simulink model "boot_demo"  (Simulink 7.3)
settings: Solver=FixedStepDiscrete  SolverMode=SingleTasking  StartTime=0.0  StopTime=10.0  RelTol=1e-3
PreLoadFcn:
  | waijung.modelPreload; % Required for working with Waijung Blockset. Do not remove.
undefined symbols (not defined in the file): HSEOSC, Link, LQFP176, ST, STM32F417IG
libraries: simulink x43, stm32f4_flash_lib x14, waijung_filestream_lib x4, stm32f4_crc_lib x3, stm32f4_boot_lib x2, stm32f4_io_lib x1, stm32f4_reset_lib x1, stm32f4_device_config_lib x1
CloseFcn:
  | waijung.modelClose; % Required for working with Waijung Blockset. Do not remove.
settings Model: Creator=Krisada  LastModifiedBy=Krisada
settings OptimizationCC: OptimizeModelRefInitCode=on  LifeSpan=1
settings HardwareCC: ProdEndianess=LittleEndian  ProdHWDeviceType=ARM Compatible->Cortex - M4  TargetEndianess=LittleEndian  TargetHWDeviceType=ARM Compatible->Cortex - M4
settings RTWCC: SystemTargetFile=stm32f4.tlc  GenerateMakefile=off  TemplateMakefile=ert_default_tmf  Description=STM32F4 Target  ProcessScript=stm32f4_make_rtw_hook
settings CodeAppCC: IgnoreCustomStorageClasses=off
settings STFCustomTargetCC: ModelReferenceCompliant=off  CombineOutputUpdateFcns=on  ERTCustomFileBanners=on  SupportContinuousTime=off  SupportNonInlinedSFcns=off  SystemTargetFile=stm32f4.tlc
settings ERTTargetCC: MultiwordLength=2048  ModelReferenceCompliant=off  ParMdlRefBuildCompliant=off  CompOptLevelCompliant=off  ERTFirstTimeCompliant=off  ModelStepFunctionPrototypeControlCompliant=off  CPPClassGenCompliant=off  ExtModeMexFile=noextcomm  InlinedParameterPlacement=NonHierarchical  ERTSrcFileBannerTemplate=stm32f4_code_template.cgt  ERTHdrFileBannerTemplate=stm32f4_code_template.cgt  ERTDataSrcFileTemplate=stm32f4_code_template.cgt  ERTDataHdrFileTemplate=stm32f4_code_template.cgt  ERTCustomFileTemplate=stm32f4_file_process.tlc

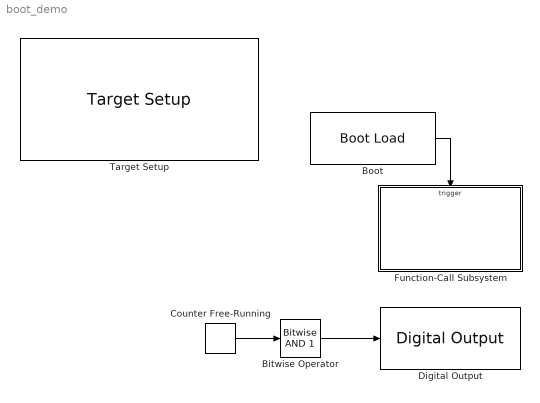
== system boot_demo ==
  Bitwise Operator : simulink/Logic and Bit Operations/Bitwise Operator  logicop=AND  UseBitMask=on  BitMask=1  BitMaskRealWorld=Stored Integer
  Boot : stm32f4_boot_lib/Boot Load  conf=Boot  flashorigin=0x8000000  flashlength=0x100000  enableisr=on  usersector=Sector 9: 0x080A0000 - 0x080BFFFF  sampletime=-1  sampletimestr=0.01  blockid=Boot  inputarray=[]  inputlabelarray={}  outputarray=[7]  outputlabelarray={'Call ISR'}  compat=0  confstr="[\"080A0000\",\"9\"]"
  Counter Free-Running : simulink/Sources/Counter Free-Running  SystemSampleTime=-1  NumBits=16  tsamp=0.5
  Digital Output : stm32f4_io_lib/Digital Output  use_bitband=on  port=D  speed=100  porttype=Push Pull  porttypestr=PP  use_pin0=off  use_pin1=off  use_pin2=off  use_pin3=off  use_pin4=off  use_pin5=off  use_pin6=off  use_pin7=off  use_pin8=off  use_pin9=off  use_pin10=off  use_pin11=off  use_pin12=off  use_pin13=off  use_pin14=off  use_pin15=on  pinstr=GPIO_Pin_15  usedpinarray="[0  0  0  0  0  0  0  0  0  0  0  0  0  0  0  1]"  bitbandingstr="#define DigitalOutput_D15 Peripheral_BB(GPIOD->ODR, 15)  /* Output pin */"  sampletime=-1  sampletimestr=0.5  blockid=DigitalOutput  enablecustomportlabel=off  globalinit=off  cinputportlabel=In1, In2  coutputportlabel=0
  Function-Call Subsystem : Subsystem  TreatAsAtomicUnit=on
  Target Setup : stm32f4_device_config_lib/Target Setup  Priority=100  compiler=GNU ARM  previous_compiler=GNU ARM  mcu=STM32F417IG (LQFP176)  mcustr=STM32F417IG  clockconfig=HSEOSC-8MHz  system_stm32f4xx_c_path=F:\trunk\targets\stm32f4_target\stm32f4\utils\system_stm32f4xx_default\STM32F40_41xxx\hseosc8mhz  showmemoryconfiguration=off  stacksize=0x2000  heapsize=0x2000  enableautocompiledownload=on  fullchiperase=on  programmerinterface=ST-Link  editctrlstr=on  compilercontrolstr=$(patsubst %, -I%, .) -mcpu=cortex-m4 -mthumb -mthumb-interwork -mfloat-abi=hard -mfpu=fpv4-sp-d16 -ffast-math -Wall -Wextra -Ofast  assemblercontrolstr=$(patsubst %, -I%, .) -mcpu=cortex-m4 -mthumb -mthumb-interwork -mfloat-abi=hard -mfpu=fpv4-sp-d16 -ffast-math -Wall -Wextra -Ofast -Wa,-amhls=$(<:.s=.lst) -D__STACK_SIZE=$(STACK_SIZE) -D__HEAP_SIZE=$(HEAP_SIZE)  linkercontrolstr=-T$(LD_SCRIPT) -g -Wl,-Map=$(MAP),--cref,--no-warn-mismatch -mcpu=cortex-m4 -mthumb -mthumb-interwork -mfloat-abi=hard -mfpu=fpv4-sp-d16 -specs=nosys.specs  runafterdownload=on  execprofile=None  profileruart=3  profilerbaud=500000  profilertxpin=D8  profilerinitstr=0.01,168000000,1680000,500000,0  manualsetsampletime=off  sampletime=0.01  blockid=TargetSetup  systickreloadvalue=1680000  hseval=8000000  lastprofileruart=3  hclk=168000000  flashorigin=0x8000000  flashlength=1024k  ramorigin=0x20000000  ramlength=128k  useextram=off
  wires:
  Boot/1 -> Function-Call Subsystem/Trigger
  Counter Free-Running/1 -> Bitwise Operator/1
  Bitwise Operator/1 -> Digital Output/1

== system boot_demo/Function-Call Subsystem ==
  function : TriggerPort  TriggerType=function-call
  Load system/conf.ini : Subsystem  TreatAsAtomicUnit=on
  Logical Operator1 : Logic  Operator=NOT  AllPortsSameDT=off  OutDataTypeMode=boolean  LogicDataType=fixdt(0, 8)  OutDataTypeStr=boolean
  System Upgrade : Subsystem
  Validate Main Program : Subsystem
  wires:
  Load system/conf.ini/1(Upgrade Enable) -> System Upgrade/Enable, Logical Operator1/1
  Load system/conf.ini/2(File) -> System Upgrade/1(File)
  Logical Operator1/1 -> Validate Main Program/Enable

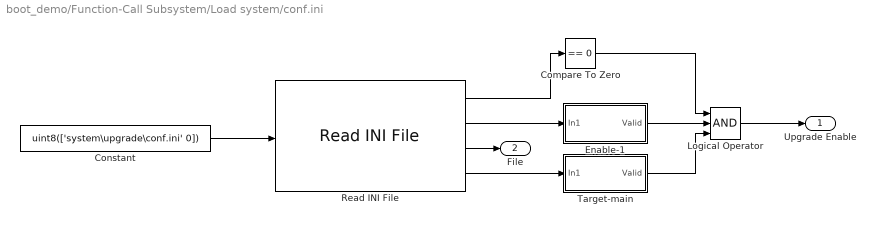
== system boot_demo/Function-Call Subsystem/Load system/conf.ini ==
  Compare To Zero : simulink/Logic and Bit Operations/Compare To Zero  SystemSampleTime=-1  relop===  LogicOutDataTypeMode=uint8  ZeroCross=off
  Constant : Constant  Value=uint8(['system\upgrade\conf.ini' 0])  OutDataType=fixdt(1, 16)  OutScaling=2^0
  Enable-1 : Subsystem
  Logical Operator : Logic  Inputs=3  AllPortsSameDT=off  OutDataTypeMode=boolean  LogicDataType=fixdt(0, 8)  OutDataTypeStr=boolean
  Read INI File : waijung_filestream_lib/Read INI File  conf=INIRead  inisection='Upgrade'  inikeys={'Enable','File','Target'}  datatype=double  datacount=1  maxstring=128  valuetype=Vector  portpinstr=0  sampletime=inf  blockid=FunctionCallSubsystemLoadsystemconfiniReadINIFile  inputporttype=[-1]  inputportwidth=[-1]  inputportlabel={'FilePath'}  outputporttype=[6 3 3 3]  outputportwidth=[1 128 128 128]  outputportlabel={'Status' 'Enable' 'File' 'Target'}  compat=0  optionstring="[\"Upgrade\",\"128\"]"  inikeylist="[\"Enable\",\"File\",\"Target\"]"
  Target-main : Subsystem
  Upgrade Enable : Outport  OutDataType=fixdt(1, 16)  OutScaling=2^0
  File : Outport  Port=2  OutDataType=fixdt(1, 16)  OutScaling=2^0
  wires:
  Constant/1 -> Read INI File/1
  Read INI File/3 -> File/1
  Read INI File/2 -> Enable-1/1(In1)
  Read INI File/4 -> Target-main/1(In1)
  Target-main/1(Valid) -> Logical Operator/3
  Enable-1/1(Valid) -> Logical Operator/2
  Read INI File/1 -> Compare To Zero/1
  Logical Operator/1 -> Upgrade Enable/1
  Compare To Zero/1 -> Logical Operator/1

== system boot_demo/Function-Call Subsystem/System Upgrade ==
  File : Inport  OutDataType=fixdt(1, 16)  OutScaling=2^0
  Enable : EnablePort
  Add : Sum  Inputs=+++  OutDataType=fixdt(1, 16)  OutScaling=2^-10
  Clear system/conf.ini : Subsystem
  Upgrade : Subsystem  TreatAsAtomicUnit=on
  Validate File : Subsystem  TreatAsAtomicUnit=on
  Verify : Subsystem  TreatAsAtomicUnit=on
  wires:
  Validate File/1(Update File Valid) -> Upgrade/Enable, Add/1
  File/1 -> Validate File/1(File), Upgrade/1(File), Clear system/conf.ini/2(File)
  Upgrade/1(Success) -> Verify/Enable, Add/2
  Verify/1(Success) -> Add/3
  Add/1 -> Clear system/conf.ini/1(Success State)

== system boot_demo/Function-Call Subsystem/Validate Main Program ==
  Enable : EnablePort
  CRC Location : Constant  Value=uint32(hex2dec('20000')-4)  OutDataType=fixdt(1, 16)  OutScaling=2^0
  Flash Read : stm32f4_flash_lib/Flash Read  conf=Read  transfer=Blocking  flashsector=Sector 7: 0x08060000 - 0x0807FFFF  datatype=uint32  datacount=1  enablestatus=off  sampletime=-1  sampletimestr=-1  blockid=FunctionCallSubsystemValidateMainProgramFlashRead  inputarray=[-1]  inputlabelarray={'Offset '}  outputarray=[7]  outputlabelarray={'Data (uint32)'}  compat=0  confstr="[\"uint32\",\"20000\",\"08060000\",\"7\",\"off\"]"
  JumpToSectorB : Subsystem  TreatAsAtomicUnit=on
  Relational Operator : RelationalOperator  Operator===  LogicOutDataTypeMode=boolean  LogicDataType=fixdt(0, 8)  OutDataTypeStr=boolean
  While Iterator Subsystem1 : Subsystem  TreatAsAtomicUnit=on
  wires:
  Flash Read/1 -> Relational Operator/1
  While Iterator Subsystem1/1(Sector CRC) -> Relational Operator/2
  CRC Location/1 -> Flash Read/1
  Relational Operator/1 -> JumpToSectorB/Enable

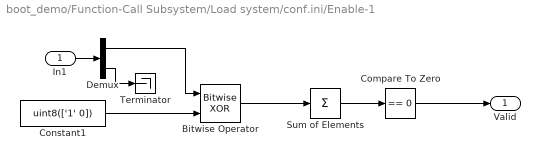
== system boot_demo/Function-Call Subsystem/Load system/conf.ini/Enable-1 ==
  In1 : Inport
  Bitwise Operator : simulink/Logic and Bit Operations/Bitwise Operator  logicop=XOR  UseBitMask=off  NumInputPorts=2  BitMask=bin2dec('11011001')  BitMaskRealWorld=Stored Integer
  Compare To Zero : simulink/Logic and Bit Operations/Compare To Zero  SystemSampleTime=-1  relop===  LogicOutDataTypeMode=uint8  ZeroCross=off
  Constant1 : Constant  Value=uint8(['1' 0])  OutDataType=fixdt(1, 16)  OutScaling=2^0
  Demux : Demux  Outputs=[2 -1]
  Sum of Elements : Sum  Inputs=+  OutDataType=fixdt(1, 16)  OutScaling=2^-10
  Terminator : Terminator
  Valid : Outport
  wires:
  In1/1 -> Demux/1
  Constant1/1 -> Bitwise Operator/2
  Bitwise Operator/1 -> Sum of Elements/1
  Sum of Elements/1 -> Compare To Zero/1
  Compare To Zero/1 -> Valid/1
  Demux/2 -> Terminator/1
  Demux/1 -> Bitwise Operator/1

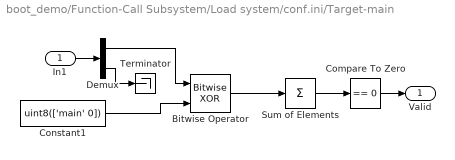
== system boot_demo/Function-Call Subsystem/Load system/conf.ini/Target-main ==
  In1 : Inport
  Bitwise Operator : simulink/Logic and Bit Operations/Bitwise Operator  logicop=XOR  UseBitMask=off  NumInputPorts=2  BitMask=bin2dec('11011001')  BitMaskRealWorld=Stored Integer
  Compare To Zero : simulink/Logic and Bit Operations/Compare To Zero  SystemSampleTime=-1  relop===  LogicOutDataTypeMode=uint8  ZeroCross=off
  Constant1 : Constant  Value=uint8(['main' 0])  OutDataType=fixdt(1, 16)  OutScaling=2^0
  Demux : Demux  Outputs=[5 -1]
  Sum of Elements : Sum  Inputs=+  OutDataType=fixdt(1, 16)  OutScaling=2^-10
  Terminator : Terminator
  Valid : Outport
  wires:
  Constant1/1 -> Bitwise Operator/2
  In1/1 -> Demux/1
  Bitwise Operator/1 -> Sum of Elements/1
  Sum of Elements/1 -> Compare To Zero/1
  Compare To Zero/1 -> Valid/1
  Demux/2 -> Terminator/1
  Demux/1 -> Bitwise Operator/1

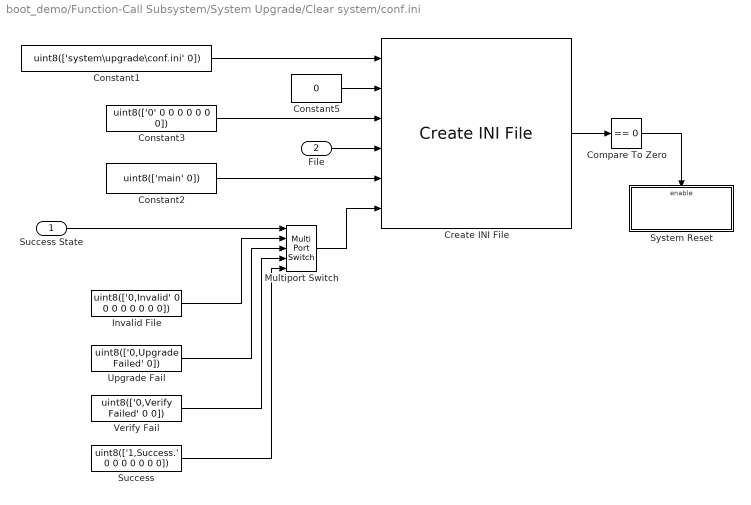
== system boot_demo/Function-Call Subsystem/System Upgrade/Clear system/conf.ini ==
  Success State : Inport  OutDataType=fixdt(1, 16)  OutScaling=2^0
  File : Inport  Port=2  OutDataType=fixdt(1, 16)  OutScaling=2^0
  Compare To Zero : simulink/Logic and Bit Operations/Compare To Zero  SystemSampleTime=-1  relop===  LogicOutDataTypeMode=uint8  ZeroCross=off
  Constant1 : Constant  Value=uint8(['system\upgrade\conf.ini' 0])  OutDataType=fixdt(1, 16)  OutScaling=2^0
  Constant2 : Constant  Value=uint8(['main' 0])  OutDataType=fixdt(1, 16)  OutScaling=2^0
  Constant3 : Constant  Value=uint8(['0' 0 0 0 0 0 0 0])  OutDataType=fixdt(1, 16)  OutScaling=2^0
  Constant5 : Constant  Value=0  OutDataType=fixdt(1, 16)  OutScaling=2^0
  Create INI File : waijung_filestream_lib/Create INI File  conf=INICreate  inisection='Upgrade'  inikeys={'Enable','File','Target','Status'}  datatype=double  datacount=1  maxstring=32  valuetype=Pointer  portpinstr=0  sampletime=inf  blockid=FunctionCallSubsystemSystemUpgradeClearsystemconfiniCreateINIFile  inputporttype=[-1 -1 -1 -1 -1 -1]  inputportwidth=[-1 1 -1 -1 -1 -1]  inputportlabel={'FilePath','Append' 'Enable' 'File' 'Target' 'Status'}  outputporttype=[6]  outputportwidth=[]  outputportlabel={'Status'}  compat=0  optionstring="[\"Upgrade\",\"32\"]"  inikeylist="[\"Enable\",\"File\",\"Target\",\"Status\"]"
  Invalid File : Constant  Value=uint8(['0,Invalid' 0 0 0 0 0 0 0 0])  OutDataType=fixdt(1, 16)  OutScaling=2^0
  Multiport Switch : MultiPortSwitch  Inputs=4  zeroidx=on  OutDataType=fixdt(1, 16)  OutScaling=2^0
  Success : Constant  Value=uint8(['1,Success.' 0 0 0 0 0 0 0])  OutDataType=fixdt(1, 16)  OutScaling=2^0
  System Reset : Subsystem  TreatAsAtomicUnit=on
  Upgrade Fail : Constant  Value=uint8(['0,Upgrade Failed' 0])  OutDataType=fixdt(1, 16)  OutScaling=2^0
  Verify Fail : Constant  Value=uint8(['0,Verify Failed' 0 0])  OutDataType=fixdt(1, 16)  OutScaling=2^0
  wires:
  Constant3/1 -> Create INI File/3
  Constant1/1 -> Create INI File/1
  Create INI File/1 -> Compare To Zero/1
  Compare To Zero/1 -> System Reset/Enable
  Success State/1 -> Multiport Switch/1
  Multiport Switch/1 -> Create INI File/6
  Constant2/1 -> Create INI File/5
  File/1 -> Create INI File/4
  Constant5/1 -> Create INI File/2
  Invalid File/1 -> Multiport Switch/2
  Upgrade Fail/1 -> Multiport Switch/3
  Verify Fail/1 -> Multiport Switch/4
  Success/1 -> Multiport Switch/5

== system boot_demo/Function-Call Subsystem/System Upgrade/Upgrade ==
  File : Inport  OutDataType=fixdt(1, 16)  OutScaling=2^0
  Enable : EnablePort
  Copy New Program : Subsystem  TreatAsAtomicUnit=on
  Erase Main Program Sector : Subsystem
  Success : Outport  OutDataType=fixdt(1, 16)  OutScaling=2^0
  wires:
  Erase Main Program Sector/1(Erased) -> Copy New Program/Enable
  File/1 -> Copy New Program/1(File)
  Copy New Program/1(Success) -> Success/1

== system boot_demo/Function-Call Subsystem/System Upgrade/Validate File ==
  File : Inport  OutDataType=fixdt(1, 16)  OutScaling=2^0
  Logical Operator : Logic  AllPortsSameDT=off  OutDataTypeMode=boolean  LogicDataType=fixdt(0, 8)  OutDataTypeStr=boolean
  Relational Operator : RelationalOperator  Operator===  LogicOutDataTypeMode=boolean  LogicDataType=fixdt(0, 8)  OutDataTypeStr=boolean
  While Iterator Subsystem : Subsystem  TreatAsAtomicUnit=on
  Update File Valid : Outport  OutDataType=fixdt(1, 16)  OutScaling=2^0
  wires:
  File/1 -> While Iterator Subsystem/1(File)
  While Iterator Subsystem/2(File CRC) -> Relational Operator/1
  While Iterator Subsystem/3(Emb CRC) -> Relational Operator/2
  Relational Operator/1 -> Logical Operator/2
  While Iterator Subsystem/1(Success) -> Logical Operator/1
  Logical Operator/1 -> Update File Valid/1

== system boot_demo/Function-Call Subsystem/System Upgrade/Verify ==
  Enable : EnablePort
  CRC Location : Constant  Value=uint32(hex2dec('20000')-4)  OutDataType=fixdt(1, 16)  OutScaling=2^0
  Flash Read : stm32f4_flash_lib/Flash Read  conf=Read  transfer=Blocking  flashsector=Sector 7: 0x08060000 - 0x0807FFFF  datatype=uint32  datacount=1  enablestatus=off  sampletime=-1  sampletimestr=-1  blockid=FunctionCallSubsystemSystemUpgradeVerifyFlashRead  inputarray=[-1]  inputlabelarray={'Offset '}  outputarray=[7]  outputlabelarray={'Data (uint32)'}  compat=0  confstr="[\"uint32\",\"20000\",\"08060000\",\"7\",\"off\"]"
  Relational Operator : RelationalOperator  Operator===  LogicOutDataTypeMode=boolean  LogicDataType=fixdt(0, 8)  OutDataTypeStr=boolean
  While Iterator Subsystem1 : Subsystem  TreatAsAtomicUnit=on
  Success : Outport  OutDataType=fixdt(1, 16)  OutScaling=2^0
  wires:
  Flash Read/1 -> Relational Operator/1
  While Iterator Subsystem1/1(Sector CRC) -> Relational Operator/2
  CRC Location/1 -> Flash Read/1
  Relational Operator/1 -> Success/1

== system boot_demo/Function-Call Subsystem/Validate Main Program/JumpToSectorB ==
  Enable : EnablePort
  Boot : stm32f4_boot_lib/Jump Sector  conf=Goto  flashorigin=0x8000000  flashlength=0x100000  enableisr=off  usersector=Sector 5: 0x08020000 - 0x0803FFFF  sampletime=inf  sampletimestr=-1  blockid=FunctionCallSubsystemValidateMainProgramJumpToSectorBBoot  inputarray=[]  inputlabelarray={}  outputarray=[]  outputlabelarray={}  compat=0  confstr="[\"08020000\",\"5\"]"

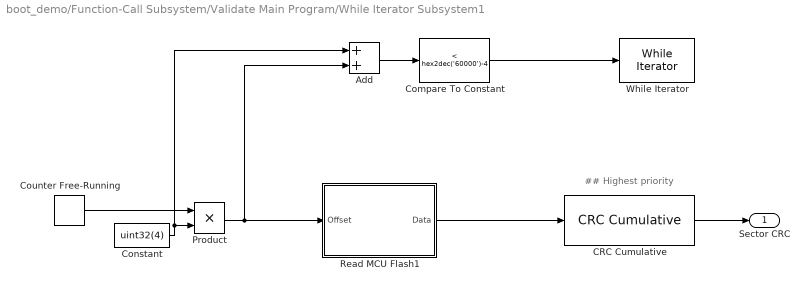
== system boot_demo/Function-Call Subsystem/Validate Main Program/While Iterator Subsystem1 ==
  note: ## Highest priority
  Add : Sum  OutDataType=fixdt(1, 16)  OutScaling=2^-10
  CRC Cumulative : stm32f4_crc_lib/CRC Cumulative  Priority=0  conf=Cumulative  sampletime=-1  sampletimestr=-1  blockid=FunctionCallSubsystemValidateMainProgramWhileIteratorSubsystem1CRCCumulative  inputarray=[7]  inputlabelarray={'uint32'}  outputarray=[7]  outputlabelarray={'uint32'}  compat=0  confstr="[\"Param1\",\"Param1\"]"
  Compare To Constant : simulink/Logic and Bit Operations/Compare To Constant  SystemSampleTime=-1  relop=<  const=hex2dec('60000')-4  LogicOutDataTypeMode=uint8  ZeroCross=off
  Constant : Constant  Value=uint32(4)  OutDataType=fixdt(1, 16)  OutScaling=2^0
  Counter Free-Running : simulink/Sources/Counter Free-Running  SystemSampleTime=-1  NumBits=32  tsamp=-1
  Product : Product  OutDataTypeMode=uint32  OutDataType=fixdt(1, 16)  OutScaling=2^0  OutDataTypeStr=uint32  RndMeth=Zero
  Read MCU Flash1 : Subsystem
  While Iterator : WhileIterator  Priority=1  MaxIters=-1  WhileBlockType=do-while
  Sector CRC : Outport  OutDataType=fixdt(1, 16)  OutScaling=2^0
  wires:
  Counter Free-Running/1 -> Product/1
  Compare To Constant/1 -> While Iterator/1
  Product/1 -> Add/2, Read MCU Flash1/1(Offset)
  Constant/1 -> Product/2, Add/1
  Read MCU Flash1/1(Data) -> CRC Cumulative/1
  CRC Cumulative/1 -> Sector CRC/1
  Add/1 -> Compare To Constant/1

== system boot_demo/Function-Call Subsystem/System Upgrade/Clear system/conf.ini/System Reset ==
  Enable : EnablePort
  System Reset : stm32f4_reset_lib/System Reset  conf=<empty>  sampletime=inf  sampletimestr=-1  blockid=FunctionCallSubsystemSystemUpgradeClearsystemconfiniSystemResetSystemReset  inputarray=[]  inputlabelarray={}  outputarray=[]  outputlabelarray={}  compat=0  confstr="[\"Param1\",\"Param1\"]"

== system boot_demo/Function-Call Subsystem/System Upgrade/Upgrade/Copy New Program ==
  File : Inport  OutDataType=fixdt(1, 16)  OutScaling=2^0
  Enable : EnablePort
  Read File-Write Flash : Subsystem  TreatAsAtomicUnit=on
  Success : Outport  OutDataType=fixdt(1, 16)  OutScaling=2^0
  wires:
  File/1 -> Read File-Write Flash/1(File)
  Read File-Write Flash/1(Success) -> Success/1

== system boot_demo/Function-Call Subsystem/System Upgrade/Upgrade/Erase Main Program Sector ==
  Compare To Zero : simulink/Logic and Bit Operations/Compare To Zero  SystemSampleTime=-1  relop===  LogicOutDataTypeMode=uint8  ZeroCross=off
  Compare To Zero1 : simulink/Logic and Bit Operations/Compare To Zero  SystemSampleTime=-1  relop===  LogicOutDataTypeMode=uint8  ZeroCross=off
  Compare To Zero2 : simulink/Logic and Bit Operations/Compare To Zero  SystemSampleTime=-1  relop===  LogicOutDataTypeMode=uint8  ZeroCross=off
  Flash Erase : stm32f4_flash_lib/Flash Erase  conf=Erase  transfer=Blocking  flashsector=Sector 5: 0x08020000 - 0x0803FFFF  datatype=uint32  datacount=1  enablestatus=on  sampletime=-1  sampletimestr=-1  blockid=FunctionCallSubsystemSystemUpgradeUpgradeEraseMainProgramSectorFlashErase  inputarray=[]  inputlabelarray={}  outputarray=[3]  outputlabelarray={'Status'}  compat=0  confstr="[\"Blocking\",\"on\",\"08020000\",\"5\"]"
  Flash Erase1 : stm32f4_flash_lib/Flash Erase  conf=Erase  transfer=Blocking  flashsector=Sector 6: 0x08040000 - 0x0805FFFF  datatype=uint32  datacount=1  enablestatus=on  sampletime=-1  sampletimestr=-1  blockid=FunctionCallSubsystemSystemUpgradeUpgradeEraseMainProgramSectorFlashErase1  inputarray=[]  inputlabelarray={}  outputarray=[3]  outputlabelarray={'Status'}  compat=0  confstr="[\"Blocking\",\"on\",\"08040000\",\"6\"]"
  Flash Erase2 : stm32f4_flash_lib/Flash Erase  conf=Erase  transfer=Blocking  flashsector=Sector 7: 0x08060000 - 0x0807FFFF  datatype=uint32  datacount=1  enablestatus=on  sampletime=-1  sampletimestr=-1  blockid=FunctionCallSubsystemSystemUpgradeUpgradeEraseMainProgramSectorFlashErase2  inputarray=[]  inputlabelarray={}  outputarray=[3]  outputlabelarray={'Status'}  compat=0  confstr="[\"Blocking\",\"on\",\"08060000\",\"7\"]"
  Logical Operator : Logic  Inputs=3  AllPortsSameDT=off  OutDataTypeMode=boolean  LogicDataType=fixdt(0, 8)  OutDataTypeStr=boolean
  Erased : Outport  OutDataType=fixdt(1, 16)  OutScaling=2^0
  wires:
  Flash Erase/1 -> Compare To Zero/1
  Flash Erase1/1 -> Compare To Zero1/1
  Flash Erase2/1 -> Compare To Zero2/1
  Compare To Zero1/1 -> Logical Operator/2
  Compare To Zero/1 -> Logical Operator/1
  Compare To Zero2/1 -> Logical Operator/3
  Logical Operator/1 -> Erased/1

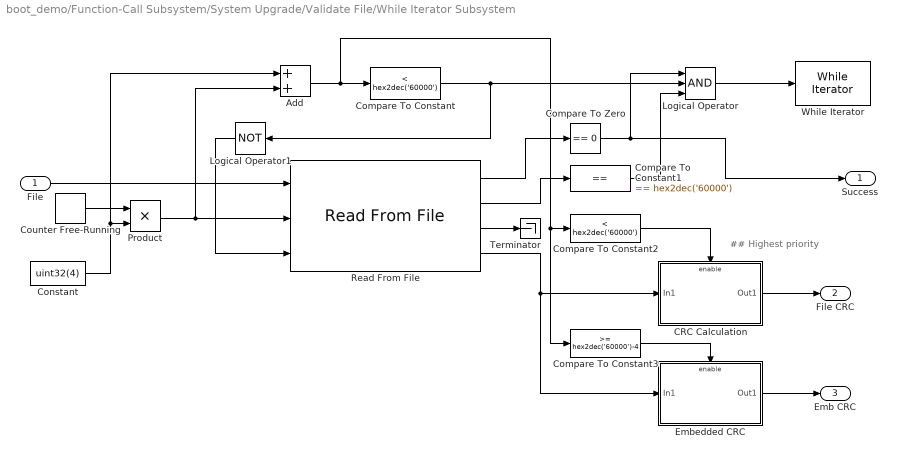
== system boot_demo/Function-Call Subsystem/System Upgrade/Validate File/While Iterator Subsystem ==
  note: ## Highest priority
  File : Inport  OutDataType=fixdt(1, 16)  OutScaling=2^0
  Add : Sum  OutDataType=fixdt(1, 16)  OutScaling=2^-10
  CRC Calculation : Subsystem
  Compare To Constant : simulink/Logic and Bit Operations/Compare To Constant  SystemSampleTime=-1  relop=<  const=hex2dec('60000')  LogicOutDataTypeMode=uint8  ZeroCross=off
  Compare To Constant1 : simulink/Logic and Bit Operations/Compare To Constant  SystemSampleTime=-1  relop===  const=hex2dec('60000')  LogicOutDataTypeMode=uint8  ZeroCross=off
  Compare To Constant2 : simulink/Logic and Bit Operations/Compare To Constant  SystemSampleTime=-1  relop=<  const=hex2dec('60000')  LogicOutDataTypeMode=uint8  ZeroCross=off
  Compare To Constant3 : simulink/Logic and Bit Operations/Compare To Constant  SystemSampleTime=-1  relop=>=  const=hex2dec('60000')-4  LogicOutDataTypeMode=uint8  ZeroCross=off
  Compare To Zero : simulink/Logic and Bit Operations/Compare To Zero  SystemSampleTime=-1  relop===  LogicOutDataTypeMode=uint8  ZeroCross=off
  Constant : Constant  Value=uint32(4)  OutDataType=fixdt(1, 16)  OutScaling=2^0
  Counter Free-Running : simulink/Sources/Counter Free-Running  SystemSampleTime=-1  NumBits=32  tsamp=-1
  Embedded CRC : Subsystem
  Logical Operator : Logic  Inputs=3  AllPortsSameDT=off  OutDataTypeMode=boolean  LogicDataType=fixdt(0, 8)  OutDataTypeStr=boolean
  Logical Operator1 : Logic  Operator=NOT  AllPortsSameDT=off  OutDataTypeMode=boolean  LogicDataType=fixdt(0, 8)  OutDataTypeStr=boolean
  Product : Product  OutDataTypeMode=uint32  OutDataType=fixdt(1, 16)  OutScaling=2^0  OutDataTypeStr=uint32  RndMeth=Zero
  Read From File : waijung_filestream_lib/Read From File  conf=ReadFromFile  inisection='Boot'  inikeys={'Action','File'}  datatype=uint32  datacount=1  maxstring=32  valuetype=Pointer  portpinstr=0  sampletime=inf  blockid=FunctionCallSubsystemSystemUpgradeValidateFileWhileIteratorSubsystemReadFromFile  inputporttype=[-1 -1 -1]  inputportwidth=[-1 1 1]  inputportlabel={'FilePath','SeekPos','Close'}  outputporttype=[6 7 7 7]  outputportwidth=[1 1 1 1]  outputportlabel={'Status','TotalSize','CurrentPos','Data (uint32)'}  compat=0  optionstring="[\"Boot\",\"32\"]"  inikeylist="[\"Action\",\"File\"]"
  Terminator : Terminator
  While Iterator : WhileIterator  Priority=1  MaxIters=-1  WhileBlockType=do-while
  Success : Outport  OutDataType=fixdt(1, 16)  OutScaling=2^0
  File CRC : Outport  Port=2  OutDataType=fixdt(1, 16)  OutScaling=2^0
  Emb CRC : Outport  Port=3  OutDataType=fixdt(1, 16)  OutScaling=2^0
  wires:
  Counter Free-Running/1 -> Product/1
  Constant/1 -> Product/2, Add/1
  CRC Calculation/1(Out1) -> File CRC/1
  Add/1 -> Compare To Constant/1, Compare To Constant2/1, Compare To Constant3/1
  Read From File/4 -> CRC Calculation/1(In1), Embedded CRC/1(In1)
  File/1 -> Read From File/1
  Read From File/2 -> Compare To Constant1/1
  Read From File/1 -> Compare To Zero/1
  Logical Operator/1 -> While Iterator/1
  Compare To Constant/1 -> Logical Operator/2, Logical Operator1/1
  Compare To Zero/1 -> Logical Operator/1, Success/1
  Compare To Constant1/1 -> Logical Operator/3
  Read From File/3 -> Terminator/1
  Product/1 -> Read From File/2, Add/2
  Compare To Constant2/1 -> CRC Calculation/Enable
  Compare To Constant3/1 -> Embedded CRC/Enable
  Embedded CRC/1(Out1) -> Emb CRC/1
  Logical Operator1/1 -> Read From File/3

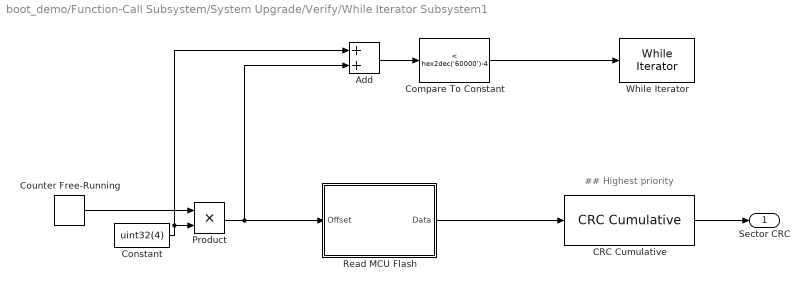
== system boot_demo/Function-Call Subsystem/System Upgrade/Verify/While Iterator Subsystem1 ==
  note: ## Highest priority
  Add : Sum  OutDataType=fixdt(1, 16)  OutScaling=2^-10
  CRC Cumulative : stm32f4_crc_lib/CRC Cumulative  Priority=0  conf=Cumulative  sampletime=-1  sampletimestr=-1  blockid=FunctionCallSubsystemSystemUpgradeVerifyWhileIteratorSubsystem1CRCCumulative  inputarray=[7]  inputlabelarray={'uint32'}  outputarray=[7]  outputlabelarray={'uint32'}  compat=0  confstr="[\"Param1\",\"Param1\"]"
  Compare To Constant : simulink/Logic and Bit Operations/Compare To Constant  SystemSampleTime=-1  relop=<  const=hex2dec('60000')-4  LogicOutDataTypeMode=uint8  ZeroCross=off
  Constant : Constant  Value=uint32(4)  OutDataType=fixdt(1, 16)  OutScaling=2^0
  Counter Free-Running : simulink/Sources/Counter Free-Running  SystemSampleTime=-1  NumBits=32  tsamp=-1
  Product : Product  OutDataTypeMode=uint32  OutDataType=fixdt(1, 16)  OutScaling=2^0  OutDataTypeStr=uint32  RndMeth=Zero
  Read MCU Flash : Subsystem
  While Iterator : WhileIterator  Priority=1  MaxIters=-1  WhileBlockType=do-while
  Sector CRC : Outport  OutDataType=fixdt(1, 16)  OutScaling=2^0
  wires:
  Counter Free-Running/1 -> Product/1
  Compare To Constant/1 -> While Iterator/1
  Product/1 -> Add/2, Read MCU Flash/1(Offset)
  Constant/1 -> Product/2, Add/1
  Read MCU Flash/1(Data) -> CRC Cumulative/1
  CRC Cumulative/1 -> Sector CRC/1
  Add/1 -> Compare To Constant/1

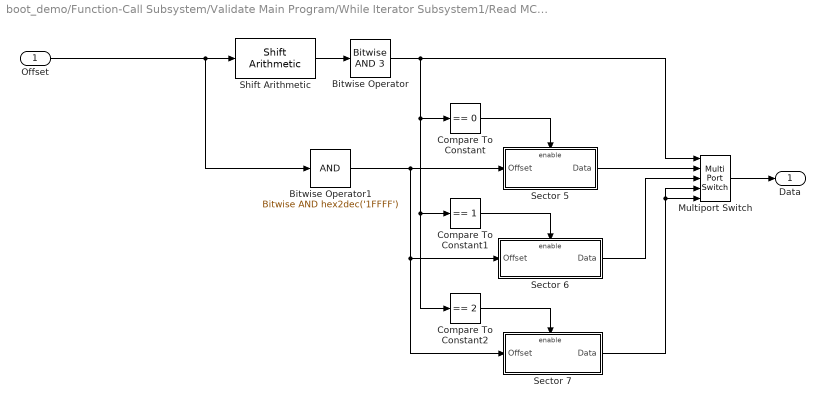
== system boot_demo/Function-Call Subsystem/Validate Main Program/While Iterator Subsystem1/Read MCU Flash1 ==
  Offset : Inport
  Bitwise Operator : simulink/Logic and Bit Operations/Bitwise Operator  logicop=AND  UseBitMask=on  BitMask=3  BitMaskRealWorld=Stored Integer
  Bitwise Operator1 : simulink/Logic and Bit Operations/Bitwise Operator  logicop=AND  UseBitMask=on  BitMask=hex2dec('1FFFF')  BitMaskRealWorld=Stored Integer
  Compare To Constant : simulink/Logic and Bit Operations/Compare To Constant  SystemSampleTime=-1  relop===  const=0  LogicOutDataTypeMode=uint8  ZeroCross=off
  Compare To Constant1 : simulink/Logic and Bit Operations/Compare To Constant  SystemSampleTime=-1  relop===  const=1  LogicOutDataTypeMode=uint8  ZeroCross=off
  Compare To Constant2 : simulink/Logic and Bit Operations/Compare To Constant  SystemSampleTime=-1  relop===  const=2  LogicOutDataTypeMode=uint8  ZeroCross=off
  Multiport Switch : MultiPortSwitch  Inputs=4  zeroidx=on  OutDataType=fixdt(1, 16)  OutScaling=2^0
  Sector 5 : Subsystem  TreatAsAtomicUnit=on
  Sector 6 : Subsystem  TreatAsAtomicUnit=on
  Sector 7 : Subsystem  TreatAsAtomicUnit=on
  Shift Arithmetic : simulink/Logic and Bit Operations/Shift Arithmetic  SystemSampleTime=-1  nBitShiftRight=17  nBinPtShiftRight=0
  Data : Outport
  wires:
  Sector 7/1(Data) -> Multiport Switch/5, Multiport Switch/4
  Sector 6/1(Data) -> Multiport Switch/3
  Bitwise Operator1/1 -> Sector 7/1(Offset), Sector 6/1(Offset), Sector 5/1(Offset)
  Offset/1 -> Bitwise Operator1/1, Shift Arithmetic/1
  Multiport Switch/1 -> Data/1
  Sector 5/1(Data) -> Multiport Switch/2
  Compare To Constant2/1 -> Sector 7/Enable
  Compare To Constant1/1 -> Sector 6/Enable
  Compare To Constant/1 -> Sector 5/Enable
  Bitwise Operator/1 -> Multiport Switch/1, Compare To Constant2/1, Compare To Constant1/1, Compare To Constant/1
  Shift Arithmetic/1 -> Bitwise Operator/1

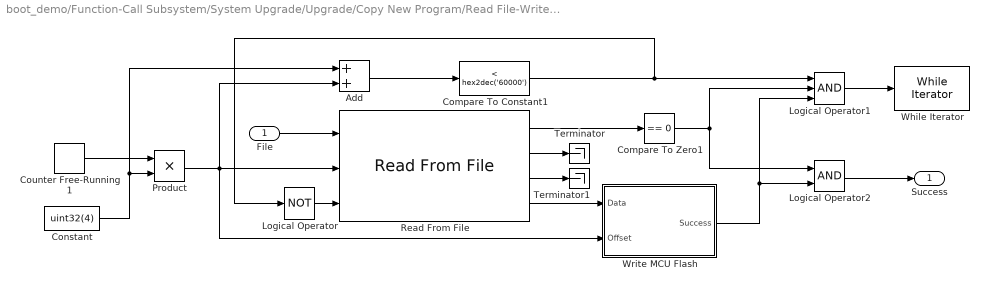
== system boot_demo/Function-Call Subsystem/System Upgrade/Upgrade/Copy New Program/Read File-Write Flash ==
  File : Inport  OutDataType=fixdt(1, 16)  OutScaling=2^0
  Add : Sum  OutDataType=fixdt(1, 16)  OutScaling=2^-10
  Compare To Constant1 : simulink/Logic and Bit Operations/Compare To Constant  SystemSampleTime=-1  relop=<  const=hex2dec('60000')  LogicOutDataTypeMode=uint8  ZeroCross=off
  Compare To Zero1 : simulink/Logic and Bit Operations/Compare To Zero  SystemSampleTime=-1  relop===  LogicOutDataTypeMode=uint8  ZeroCross=off
  Constant : Constant  Value=uint32(4)  OutDataType=fixdt(1, 16)  OutScaling=2^0
  Counter Free-Running1 : simulink/Sources/Counter Free-Running  SystemSampleTime=-1  NumBits=32  tsamp=-1
  Logical Operator : Logic  Operator=NOT  AllPortsSameDT=off  OutDataTypeMode=boolean  LogicDataType=fixdt(0, 8)  OutDataTypeStr=boolean
  Logical Operator1 : Logic  Inputs=3  AllPortsSameDT=off  OutDataTypeMode=boolean  LogicDataType=fixdt(0, 8)  OutDataTypeStr=boolean
  Logical Operator2 : Logic  AllPortsSameDT=off  OutDataTypeMode=boolean  LogicDataType=fixdt(0, 8)  OutDataTypeStr=boolean
  Product : Product  OutDataTypeMode=uint32  OutDataType=fixdt(1, 16)  OutScaling=2^0  OutDataTypeStr=uint32  RndMeth=Zero
  Read From File : waijung_filestream_lib/Read From File  conf=ReadFromFile  inisection='Boot'  inikeys={'Action','File'}  datatype=uint32  datacount=1  maxstring=32  valuetype=Pointer  portpinstr=0  sampletime=inf  blockid=FunctionCallSubsystemSystemUpgradeUpgradeCopyNewProgramReadFileWriteFlashReadFromFile  inputporttype=[-1 -1 -1]  inputportwidth=[-1 1 1]  inputportlabel={'FilePath','SeekPos','Close'}  outputporttype=[6 7 7 7]  outputportwidth=[1 1 1 1]  outputportlabel={'Status','TotalSize','CurrentPos','Data (uint32)'}  compat=0  optionstring="[\"Boot\",\"32\"]"  inikeylist="[\"Action\",\"File\"]"
  Terminator : Terminator
  Terminator1 : Terminator
  While Iterator : WhileIterator  MaxIters=-1  WhileBlockType=do-while
  Write MCU Flash : Subsystem
  Success : Outport  OutDataType=fixdt(1, 16)  OutScaling=2^0
  wires:
  Logical Operator1/1 -> While Iterator/1
  Compare To Constant1/1 -> Logical Operator1/1, Logical Operator/1
  Add/1 -> Compare To Constant1/1
  Constant/1 -> Add/1, Product/2
  Product/1 -> Add/2, Read From File/2, Write MCU Flash/2(Offset)
  Counter Free-Running1/1 -> Product/1
  File/1 -> Read From File/1
  Logical Operator/1 -> Read From File/3
  Read From File/1 -> Compare To Zero1/1
  Compare To Zero1/1 -> Logical Operator1/2, Logical Operator2/1
  Read From File/4 -> Write MCU Flash/1(Data)
  Logical Operator2/1 -> Success/1
  Read From File/2 -> Terminator/1
  Read From File/3 -> Terminator1/1
  Write MCU Flash/1(Success) -> Logical Operator2/2, Logical Operator1/3

== system boot_demo/Function-Call Subsystem/System Upgrade/Validate File/While Iterator Subsystem/CRC Calculation ==
  In1 : Inport
  Enable : EnablePort
  CRC Cumulative : stm32f4_crc_lib/CRC Cumulative  Priority=0  conf=Cumulative  sampletime=-1  sampletimestr=-1  blockid=FunctionCallSubsystemSystemUpgradeValidateFileWhileIteratorSubsystemCRCCalculationCRCCumulative  inputarray=[7]  inputlabelarray={'uint32'}  outputarray=[7]  outputlabelarray={'uint32'}  compat=0  confstr="[\"Param1\",\"Param1\"]"
  Out1 : Outport
  wires:
  In1/1 -> CRC Cumulative/1
  CRC Cumulative/1 -> Out1/1

== system boot_demo/Function-Call Subsystem/System Upgrade/Validate File/While Iterator Subsystem/Embedded CRC ==
  In1 : Inport
  Enable : EnablePort
  Out1 : Outport
  wires:
  In1/1 -> Out1/1

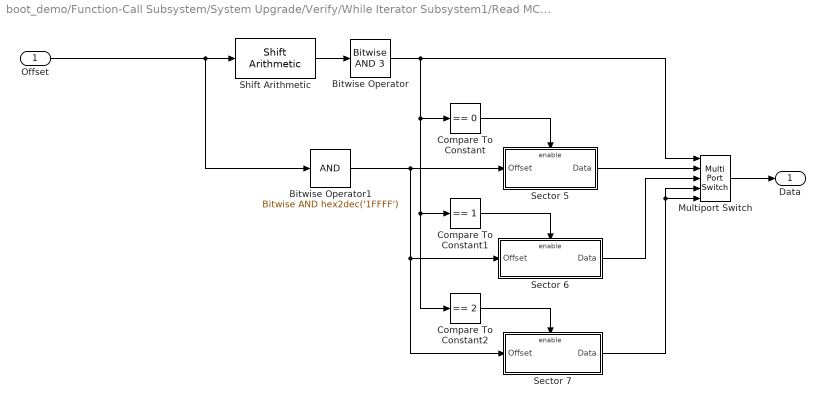
== system boot_demo/Function-Call Subsystem/System Upgrade/Verify/While Iterator Subsystem1/Read MCU Flash ==
  Offset : Inport
  Bitwise Operator : simulink/Logic and Bit Operations/Bitwise Operator  logicop=AND  UseBitMask=on  BitMask=3  BitMaskRealWorld=Stored Integer
  Bitwise Operator1 : simulink/Logic and Bit Operations/Bitwise Operator  logicop=AND  UseBitMask=on  BitMask=hex2dec('1FFFF')  BitMaskRealWorld=Stored Integer
  Compare To Constant : simulink/Logic and Bit Operations/Compare To Constant  SystemSampleTime=-1  relop===  const=0  LogicOutDataTypeMode=uint8  ZeroCross=off
  Compare To Constant1 : simulink/Logic and Bit Operations/Compare To Constant  SystemSampleTime=-1  relop===  const=1  LogicOutDataTypeMode=uint8  ZeroCross=off
  Compare To Constant2 : simulink/Logic and Bit Operations/Compare To Constant  SystemSampleTime=-1  relop===  const=2  LogicOutDataTypeMode=uint8  ZeroCross=off
  Multiport Switch : MultiPortSwitch  Inputs=4  zeroidx=on  OutDataType=fixdt(1, 16)  OutScaling=2^0
  Sector 5 : Subsystem  TreatAsAtomicUnit=on
  Sector 6 : Subsystem  TreatAsAtomicUnit=on
  Sector 7 : Subsystem  TreatAsAtomicUnit=on
  Shift Arithmetic : simulink/Logic and Bit Operations/Shift Arithmetic  SystemSampleTime=-1  nBitShiftRight=17  nBinPtShiftRight=0
  Data : Outport
  wires:
  Shift Arithmetic/1 -> Bitwise Operator/1
  Bitwise Operator/1 -> Compare To Constant/1, Compare To Constant1/1, Compare To Constant2/1, Multiport Switch/1
  Compare To Constant/1 -> Sector 5/Enable
  Compare To Constant1/1 -> Sector 6/Enable
  Compare To Constant2/1 -> Sector 7/Enable
  Sector 5/1(Data) -> Multiport Switch/2
  Multiport Switch/1 -> Data/1
  Offset/1 -> Shift Arithmetic/1, Bitwise Operator1/1
  Bitwise Operator1/1 -> Sector 5/1(Offset), Sector 6/1(Offset), Sector 7/1(Offset)
  Sector 6/1(Data) -> Multiport Switch/3
  Sector 7/1(Data) -> Multiport Switch/4, Multiport Switch/5

== system boot_demo/Function-Call Subsystem/Validate Main Program/While Iterator Subsystem1/Read MCU Flash1/Sector 5 ==
  Offset : Inport  OutDataType=fixdt(1, 16)  OutScaling=2^0
  Enable : EnablePort
  Flash Read : stm32f4_flash_lib/Flash Read  conf=Read  transfer=Blocking  flashsector=Sector 5: 0x08020000 - 0x0803FFFF  datatype=uint32  datacount=1  enablestatus=on  sampletime=-1  sampletimestr=-1  blockid=FunctionCallSubsystemValidateMainProgramWhileIteratorSubsystem1ReadMCUFlash1Sector5FlashRead  inputarray=[-1]  inputlabelarray={'Offset '}  outputarray=[7]  outputlabelarray={'Data (uint32)'}  compat=0  confstr="[\"uint32\",\"20000\",\"08020000\",\"5\",\"on\"]"
  Data : Outport  OutDataType=fixdt(1, 16)  OutScaling=2^0
  wires:
  Flash Read/1 -> Data/1
  Offset/1 -> Flash Read/1

== system boot_demo/Function-Call Subsystem/Validate Main Program/While Iterator Subsystem1/Read MCU Flash1/Sector 6 ==
  Offset : Inport  OutDataType=fixdt(1, 16)  OutScaling=2^0
  Enable : EnablePort
  Flash Read : stm32f4_flash_lib/Flash Read  conf=Read  transfer=Blocking  flashsector=Sector 6: 0x08040000 - 0x0805FFFF  datatype=uint32  datacount=1  enablestatus=on  sampletime=-1  sampletimestr=-1  blockid=FunctionCallSubsystemValidateMainProgramWhileIteratorSubsystem1ReadMCUFlash1Sector6FlashRead  inputarray=[-1]  inputlabelarray={'Offset '}  outputarray=[7]  outputlabelarray={'Data (uint32)'}  compat=0  confstr="[\"uint32\",\"20000\",\"08040000\",\"6\",\"on\"]"
  Data : Outport  OutDataType=fixdt(1, 16)  OutScaling=2^0
  wires:
  Offset/1 -> Flash Read/1
  Flash Read/1 -> Data/1

== system boot_demo/Function-Call Subsystem/Validate Main Program/While Iterator Subsystem1/Read MCU Flash1/Sector 7 ==
  Offset : Inport  OutDataType=fixdt(1, 16)  OutScaling=2^0
  Enable : EnablePort
  Flash Read : stm32f4_flash_lib/Flash Read  conf=Read  transfer=Blocking  flashsector=Sector 7: 0x08060000 - 0x0807FFFF  datatype=uint32  datacount=1  enablestatus=on  sampletime=-1  sampletimestr=-1  blockid=FunctionCallSubsystemValidateMainProgramWhileIteratorSubsystem1ReadMCUFlash1Sector7FlashRead  inputarray=[-1]  inputlabelarray={'Offset '}  outputarray=[7]  outputlabelarray={'Data (uint32)'}  compat=0  confstr="[\"uint32\",\"20000\",\"08060000\",\"7\",\"on\"]"
  Data : Outport  OutDataType=fixdt(1, 16)  OutScaling=2^0
  wires:
  Offset/1 -> Flash Read/1
  Flash Read/1 -> Data/1

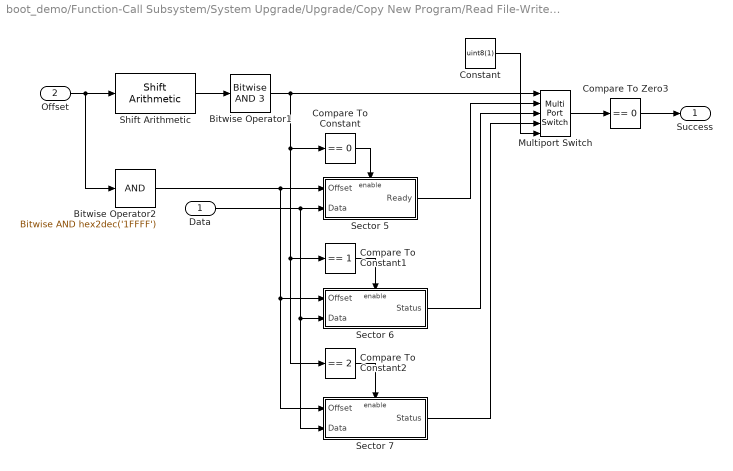
== system boot_demo/Function-Call Subsystem/System Upgrade/Upgrade/Copy New Program/Read File-Write Flash/Write MCU Flash ==
  Data : Inport
  Offset : Inport  Port=2
  Bitwise Operator1 : simulink/Logic and Bit Operations/Bitwise Operator  logicop=AND  UseBitMask=on  BitMask=3  BitMaskRealWorld=Stored Integer
  Bitwise Operator2 : simulink/Logic and Bit Operations/Bitwise Operator  logicop=AND  UseBitMask=on  BitMask=hex2dec('1FFFF')  BitMaskRealWorld=Stored Integer
  Compare To Constant : simulink/Logic and Bit Operations/Compare To Constant  SystemSampleTime=-1  relop===  const=0  LogicOutDataTypeMode=uint8  ZeroCross=off
  Compare To Constant1 : simulink/Logic and Bit Operations/Compare To Constant  SystemSampleTime=-1  relop===  const=1  LogicOutDataTypeMode=uint8  ZeroCross=off
  Compare To Constant2 : simulink/Logic and Bit Operations/Compare To Constant  SystemSampleTime=-1  relop===  const=2  LogicOutDataTypeMode=uint8  ZeroCross=off
  Compare To Zero3 : simulink/Logic and Bit Operations/Compare To Zero  SystemSampleTime=-1  relop===  LogicOutDataTypeMode=uint8  ZeroCross=off
  Constant : Constant  Value=uint8(1)  OutDataType=fixdt(1, 16)  OutScaling=2^0
  Multiport Switch : MultiPortSwitch  Inputs=4  zeroidx=on  OutDataType=fixdt(1, 16)  OutScaling=2^0
  Sector 5 : Subsystem  TreatAsAtomicUnit=on
  Sector 6 : Subsystem  TreatAsAtomicUnit=on
  Sector 7 : Subsystem  TreatAsAtomicUnit=on
  Shift Arithmetic : simulink/Logic and Bit Operations/Shift Arithmetic  SystemSampleTime=-1  nBitShiftRight=17  nBinPtShiftRight=0
  Success : Outport
  wires:
  Shift Arithmetic/1 -> Bitwise Operator1/1
  Offset/1 -> Shift Arithmetic/1, Bitwise Operator2/1
  Compare To Constant/1 -> Sector 5/Enable
  Bitwise Operator1/1 -> Compare To Constant/1, Compare To Constant1/1, Compare To Constant2/1, Multiport Switch/1
  Bitwise Operator2/1 -> Sector 5/1(Offset), Sector 6/1(Offset), Sector 7/1(Offset)
  Data/1 -> Sector 5/2(Data), Sector 6/2(Data), Sector 7/2(Data)
  Compare To Constant1/1 -> Sector 6/Enable
  Compare To Constant2/1 -> Sector 7/Enable
  Multiport Switch/1 -> Compare To Zero3/1
  Compare To Zero3/1 -> Success/1
  Sector 5/1(Ready) -> Multiport Switch/2
  Sector 6/1(Status) -> Multiport Switch/3
  Sector 7/1(Status) -> Multiport Switch/4
  Constant/1 -> Multiport Switch/5

== system boot_demo/Function-Call Subsystem/System Upgrade/Verify/While Iterator Subsystem1/Read MCU Flash/Sector 5 ==
  Offset : Inport  OutDataType=fixdt(1, 16)  OutScaling=2^0
  Enable : EnablePort
  Flash Read : stm32f4_flash_lib/Flash Read  conf=Read  transfer=Blocking  flashsector=Sector 5: 0x08020000 - 0x0803FFFF  datatype=uint32  datacount=1  enablestatus=on  sampletime=-1  sampletimestr=-1  blockid=FunctionCallSubsystemSystemUpgradeVerifyWhileIteratorSubsystem1ReadMCUFlashSector5FlashRead  inputarray=[-1]  inputlabelarray={'Offset '}  outputarray=[7]  outputlabelarray={'Data (uint32)'}  compat=0  confstr="[\"uint32\",\"20000\",\"08020000\",\"5\",\"on\"]"
  Data : Outport  OutDataType=fixdt(1, 16)  OutScaling=2^0
  wires:
  Offset/1 -> Flash Read/1
  Flash Read/1 -> Data/1

== system boot_demo/Function-Call Subsystem/System Upgrade/Verify/While Iterator Subsystem1/Read MCU Flash/Sector 6 ==
  Offset : Inport  OutDataType=fixdt(1, 16)  OutScaling=2^0
  Enable : EnablePort
  Flash Read : stm32f4_flash_lib/Flash Read  conf=Read  transfer=Blocking  flashsector=Sector 6: 0x08040000 - 0x0805FFFF  datatype=uint32  datacount=1  enablestatus=on  sampletime=-1  sampletimestr=-1  blockid=FunctionCallSubsystemSystemUpgradeVerifyWhileIteratorSubsystem1ReadMCUFlashSector6FlashRead  inputarray=[-1]  inputlabelarray={'Offset '}  outputarray=[7]  outputlabelarray={'Data (uint32)'}  compat=0  confstr="[\"uint32\",\"20000\",\"08040000\",\"6\",\"on\"]"
  Data : Outport  OutDataType=fixdt(1, 16)  OutScaling=2^0
  wires:
  Flash Read/1 -> Data/1
  Offset/1 -> Flash Read/1

== system boot_demo/Function-Call Subsystem/System Upgrade/Verify/While Iterator Subsystem1/Read MCU Flash/Sector 7 ==
  Offset : Inport  OutDataType=fixdt(1, 16)  OutScaling=2^0
  Enable : EnablePort
  Flash Read : stm32f4_flash_lib/Flash Read  conf=Read  transfer=Blocking  flashsector=Sector 7: 0x08060000 - 0x0807FFFF  datatype=uint32  datacount=1  enablestatus=on  sampletime=-1  sampletimestr=-1  blockid=FunctionCallSubsystemSystemUpgradeVerifyWhileIteratorSubsystem1ReadMCUFlashSector7FlashRead  inputarray=[-1]  inputlabelarray={'Offset '}  outputarray=[7]  outputlabelarray={'Data (uint32)'}  compat=0  confstr="[\"uint32\",\"20000\",\"08060000\",\"7\",\"on\"]"
  Data : Outport  OutDataType=fixdt(1, 16)  OutScaling=2^0
  wires:
  Flash Read/1 -> Data/1
  Offset/1 -> Flash Read/1

== system boot_demo/Function-Call Subsystem/System Upgrade/Upgrade/Copy New Program/Read File-Write Flash/Write MCU Flash/Sector 5 ==
  Offset : Inport  OutDataType=fixdt(1, 16)  OutScaling=2^0
  Data : Inport  Port=2  OutDataType=fixdt(1, 16)  OutScaling=2^0
  Enable : EnablePort
  Flash Write1 : stm32f4_flash_lib/Flash Write  conf=Program  transfer=Blocking  flashsector=Sector 5: 0x08020000 - 0x0803FFFF  datatype=uint32  datacount=1  enablestatus=on  sampletime=-1  sampletimestr=-1  blockid=FunctionCallSubsystemSystemUpgradeUpgradeCopyNewProgramReadFileWriteFlashWriteMCUFlashSector5FlashWrite1  inputarray=[-1,7]  inputlabelarray={'Offset ', 'Data (uint32)'}  outputarray=[3]  outputlabelarray={'Status'}  compat=0  confstr="[\"Blocking\",\"uint32\",\"on\",\"20000\",\"08020000\",\"5\"]"
  Ready : Outport  OutDataType=fixdt(1, 16)  OutScaling=2^0
  wires:
  Offset/1 -> Flash Write1/1
  Data/1 -> Flash Write1/2
  Flash Write1/1 -> Ready/1

== system boot_demo/Function-Call Subsystem/System Upgrade/Upgrade/Copy New Program/Read File-Write Flash/Write MCU Flash/Sector 6 ==
  Offset : Inport  OutDataType=fixdt(1, 16)  OutScaling=2^0
  Data : Inport  Port=2  OutDataType=fixdt(1, 16)  OutScaling=2^0
  Enable : EnablePort
  Flash Write1 : stm32f4_flash_lib/Flash Write  conf=Program  transfer=Blocking  flashsector=Sector 6: 0x08040000 - 0x0805FFFF  datatype=uint32  datacount=1  enablestatus=on  sampletime=-1  sampletimestr=-1  blockid=FunctionCallSubsystemSystemUpgradeUpgradeCopyNewProgramReadFileWriteFlashWriteMCUFlashSector6FlashWrite1  inputarray=[-1,7]  inputlabelarray={'Offset ', 'Data (uint32)'}  outputarray=[3]  outputlabelarray={'Status'}  compat=0  confstr="[\"Blocking\",\"uint32\",\"on\",\"20000\",\"08040000\",\"6\"]"
  Status : Outport  OutDataType=fixdt(1, 16)  OutScaling=2^0
  wires:
  Flash Write1/1 -> Status/1
  Data/1 -> Flash Write1/2
  Offset/1 -> Flash Write1/1

== system boot_demo/Function-Call Subsystem/System Upgrade/Upgrade/Copy New Program/Read File-Write Flash/Write MCU Flash/Sector 7 ==
  Offset : Inport  OutDataType=fixdt(1, 16)  OutScaling=2^0
  Data : Inport  Port=2  OutDataType=fixdt(1, 16)  OutScaling=2^0
  Enable : EnablePort
  Flash Write1 : stm32f4_flash_lib/Flash Write  conf=Program  transfer=Blocking  flashsector=Sector 7: 0x08060000 - 0x0807FFFF  datatype=uint32  datacount=1  enablestatus=on  sampletime=-1  sampletimestr=-1  blockid=FunctionCallSubsystemSystemUpgradeUpgradeCopyNewProgramReadFileWriteFlashWriteMCUFlashSector7FlashWrite1  inputarray=[-1,7]  inputlabelarray={'Offset ', 'Data (uint32)'}  outputarray=[3]  outputlabelarray={'Status'}  compat=0  confstr="[\"Blocking\",\"uint32\",\"on\",\"20000\",\"08060000\",\"7\"]"
  Status : Outport  OutDataType=fixdt(1, 16)  OutScaling=2^0
  wires:
  Data/1 -> Flash Write1/2
  Flash Write1/1 -> Status/1
  Offset/1 -> Flash Write1/1
